simulink model "FaultCheck"  (R2022b)
settings: Solver=FixedStepAuto  StartTime=0.0  StopTime=10  FixedStep=1  RelTol=1e-3
undefined symbols (not defined in the file): C_Flt_IGBTULowerTempConfirmTh_u16, C_Flt_IGBTULowerTempDiagEn_b, C_Flt_IGBTULowerTempErrCode_u16, C_Flt_IGBTULowerTempPowerCoeff, C_Flt_IGBTULowerTempRecoveryTh_u16, C_Flt_IGBTULowerTempRecTh_s32, C_Flt_IGBTULowerTempTrigTh_s32, C_Flt_IGBTUOverTempConfirmTh_u16, C_Flt_IGBTUOverTempDiagEn_b, C_Flt_IGBTUOverTempErrCode_u16, C_Flt_IGBTUOverTempRecoveryTh_u16, C_Flt_IGBTUOverTempRecTh_s32, C_Flt_IGBTUOverTempTrigTh_s32, C_Flt_IGBTVLowerTempConfirmTh_u16, C_Flt_IGBTVLowerTempDiagEn_b, C_Flt_IGBTVLowerTempErrCode_u16, C_Flt_IGBTVLowerTempPowerCoeff, C_Flt_IGBTVLowerTempRecoveryTh_u16, C_Flt_IGBTVLowerTempRecTh_s32, C_Flt_IGBTVLowerTempTrigTh_s32, C_Flt_IGBTVOverTempConfirmTh_u16, C_Flt_IGBTVOverTempDiagEn_b, C_Flt_IGBTVOverTempErrCode_u16, C_Flt_IGBTVOverTempRecoveryTh_u16, C_Flt_IGBTVOverTempRecTh_s32, C_Flt_IGBTVOverTempTrigTh_s32, C_Flt_IGBTWLowerTempConfirmTh_u16, C_Flt_IGBTWLowerTempDiagEn_b, C_Flt_IGBTWLowerTempErrCode_u16, C_Flt_IGBTWLowerTempPowerCoeff, C_Flt_IGBTWLowerTempRecoveryTh_u16, C_Flt_IGBTWLowerTempRecTh_s32, C_Flt_IGBTWLowerTempTrigTh_s32, C_Flt_IGBTWOverTempConfirmTh_u16, C_Flt_IGBTWOverTempDiagEn_b, C_Flt_IGBTWOverTempErrCode_u16, C_Flt_IGBTWOverTempRecoveryTh_u16, C_Flt_IGBTWOverTempRecTh_s32, C_Flt_IGBTWOverTempTrigTh_s32, C_Flt_IuOCConfirmTh_u16, C_Flt_IuOCDiagEn_b, C_Flt_IuOCErrCode_u16, C_Flt_IuOCNegLimit_s32, C_Flt_IuOCPosLimit_s32, C_Flt_IuOCRecoveryTh_u16, C_Flt_IuZeroDriftDiagEn_b, C_Flt_IuZeroDriftErrCode_u16, C_Flt_IvOCConfirmTh_u16, C_Flt_IvOCDiagEn_b, C_Flt_IvOCErrCode_u16, C_Flt_IvOCNegLimit_s32, C_Flt_IvOCPosLimit_s32, C_Flt_IvOCRecoveryTh_u16, C_Flt_IvZeroDriftDiagEn_b, C_Flt_IvZeroDriftErrCode_u16, C_Flt_IwOCConfirmTh_u16, C_Flt_IwOCDiagEn_b, C_Flt_IwOCErrCode_u16, C_Flt_IwOCNegLimit_s32, C_Flt_IwOCPosLimit_s32 ... (+196)
libraries: YS_UserDefined_Library x21, simulink x5
(part 9 of 11)

== system FaultCheck/FaultDiag_HighTask_100us/FltDetn/CurrentSensorDetn/Flt_CurrentSensorDetn/ErrCode/If Action Subsystem ==
  Action Port : ActionPort
  Assignment : Assignment  IndexMode=Zero-based  DiagnosticForDimensions=Warning  IndexOptions=Index vector (port)  Indices=1  OutputSizes=1
  Constant : Constant  Value=FLT_ERRCODE_0  OutDataTypeStr=fixdt('uint16', 'DataTypeOverride', 'Off')
  Constant1 : Constant  Value=FLT_ERRBIT_53
  Data Store Read : DataStoreRead  DataStoreName=Flt_ErrCode  IndexOptions=Index vector (dialog)  Indices=1  OutputSizes=1
  Data Store Write : DataStoreWrite  DataStoreName=Flt_ErrCode  IndexOptions=Index vector (dialog)  Indices=1  OutputSizes=1
  wires:
  Assignment/1 -> Data Store Write/1
  Constant/1 -> Assignment/2
  Data Store Read/1 -> Assignment/1
  Constant1/1 -> Assignment/3

== system FaultCheck/FaultDiag_HighTask_100us/FltDetn/CurrentSensorDetn/Flt_CurrentSensorDetn/ErrCode/If Action Subsystem1 ==
  ErrCod : Inport
  Action Port : ActionPort
  Assignment : Assignment  IndexMode=Zero-based  DiagnosticForDimensions=Warning  IndexOptions=Index vector (port)  Indices=1  OutputSizes=1
  Constant : Constant  Value=FLT_ERRBIT_53
  Data Store Read : DataStoreRead  DataStoreName=Flt_ErrCode  IndexOptions=Index vector (dialog)  Indices=1  OutputSizes=1
  Data Store Write : DataStoreWrite  DataStoreName=Flt_ErrCode  IndexOptions=Index vector (dialog)  Indices=1  OutputSizes=1
  wires:
  Constant/1 -> Assignment/3
  ErrCod/1 -> Assignment/2
  Assignment/1 -> Data Store Write/1
  Data Store Read/1 -> Assignment/1

== system FaultCheck/FaultDiag_HighTask_100us/FltDetn/CurrentSensorDetn/Flt_CurrentSensorDetn/ErrDetn/If Action Subsystem ==
  Action Port : ActionPort
  Constant : Constant  Value=FLT_NOERR
  Out1 : Outport
  wires:
  Constant/1 -> Out1/1

== system FaultCheck/FaultDiag_HighTask_100us/FltDetn/CurrentSensorDetn/Flt_CurrentSensorDetn/ErrDetn/If Action Subsystem1 ==
  InputVal : Inport
  ErrDeb : Inport  Port=2
  Action Port : ActionPort
  Constant3 : Constant  Value=FLT_ERR
  Debounce1 : Subsystem
  Delay1 : Delay  DelayLength=1
  Signal Conversion : SignalConversion  OverrideOpt=off
  Switch2 : Switch  Criteria=u2 > Threshold  SaturateOnIntegerOverflow=off  InputSameDT=off
  Out1 : Outport
  wires:
  Signal Conversion/1 -> Out1/1
  Delay1/1 -> Switch2/3
  Constant3/1 -> Switch2/1
  Switch2/1 -> Signal Conversion/1, Delay1/1
  Debounce1/1(ErrFlg) -> Switch2/2
  InputVal/1 -> Debounce1/1(ErrInput)
  ErrDeb/1 -> Debounce1/2(ErrDeb)

== system FaultCheck/FaultDiag_HighTask_100us/FltDetn/CurrentSensorDetn/Flt_CurrentSensorDetn/FltLvl/If Action Subsystem ==
  Action Port : ActionPort
  Constant : Constant  Value=FLTLVL_ZERO
  ValOut : Outport
  wires:
  Constant/1 -> ValOut/1

== system FaultCheck/FaultDiag_HighTask_100us/FltDetn/CurrentSensorDetn/Flt_CurrentSensorDetn/FltLvl/If Action Subsystem1 ==
  In : Inport
  Action Port : ActionPort
  ValOut : Outport
  wires:
  In/1 -> ValOut/1

== system FaultCheck/FaultDiag_HighTask_100us/FltDetn/CurrentSensorDetn/Flt_CurrentSensorDetn/Power Reduction Coefficient/If Action Subsystem ==
  Action Port : ActionPort
  Constant1 : Constant  Value=FLT_COEF_ONE
  PowRecCoefOut : Outport
  wires:
  Constant1/1 -> PowRecCoefOut/1

== system FaultCheck/FaultDiag_HighTask_100us/FltDetn/CurrentSensorDetn/Flt_CurrentSensorDetn/Power Reduction Coefficient/If Action Subsystem1 ==
  PowRecCoef : Inport
  Action Port : ActionPort
  PowRecCoefOut : Outport
  wires:
  PowRecCoef/1 -> PowRecCoefOut/1

== system FaultCheck/FaultDiag_HighTask_100us/FltDetn/CurrentSensorDetn/Flt_CurrentSensorDetn/Power Reduction Coefficient/If Action Subsystem2 ==
  Action Port : ActionPort
  Constant1 : Constant  Value=FLT_COEF_ZERO
  PowRecCoefOut : Outport
  wires:
  Constant1/1 -> PowRecCoefOut/1

== system FaultCheck/FaultDiag_HighTask_100us/FltDetn/CurrentZeroDrfDetn/CurrZeroDrfDetn/ErrCode1/If Action Subsystem ==
  Action Port : ActionPort
  Assignment : Assignment  IndexMode=Zero-based  DiagnosticForDimensions=Warning  IndexOptions=Index vector (port)  Indices=1  OutputSizes=1
  Constant : Constant  Value=FLT_ERRCODE_0
  Constant1 : Constant  Value=FLT_ERRBIT_55
  Data Store Read : DataStoreRead  DataStoreName=Flt_ErrCode  IndexOptions=Index vector (dialog)  Indices=1  OutputSizes=1
  Data Store Write : DataStoreWrite  DataStoreName=Flt_ErrCode  IndexOptions=Index vector (dialog)  Indices=1  OutputSizes=1
  wires:
  Constant1/1 -> Assignment/3
  Data Store Read/1 -> Assignment/1
  Constant/1 -> Assignment/2
  Assignment/1 -> Data Store Write/1

== system FaultCheck/FaultDiag_HighTask_100us/FltDetn/CurrentZeroDrfDetn/CurrZeroDrfDetn/ErrCode1/If Action Subsystem1 ==
  ErrCod : Inport
  Action Port : ActionPort
  Assignment : Assignment  IndexMode=Zero-based  DiagnosticForDimensions=Warning  IndexOptions=Index vector (port)  Indices=1  OutputSizes=1
  Constant : Constant  Value=FLT_ERRBIT_55
  Data Store Read : DataStoreRead  DataStoreName=Flt_ErrCode  IndexOptions=Index vector (dialog)  Indices=1  OutputSizes=1
  Data Store Write : DataStoreWrite  DataStoreName=Flt_ErrCode  IndexOptions=Index vector (dialog)  Indices=1  OutputSizes=1
  wires:
  Data Store Read/1 -> Assignment/1
  Assignment/1 -> Data Store Write/1
  ErrCod/1 -> Assignment/2
  Constant/1 -> Assignment/3

== system FaultCheck/FaultDiag_HighTask_100us/FltDetn/CurrentZeroDrfDetn/CurrZeroDrfDetn/ErrDetn/If Action Subsystem ==
  Action Port : ActionPort
  Constant : Constant  Value=FLT_NOERR
  Out1 : Outport
  wires:
  Constant/1 -> Out1/1

== system FaultCheck/FaultDiag_HighTask_100us/FltDetn/CurrentZeroDrfDetn/CurrZeroDrfDetn/ErrDetn/If Action Subsystem1 ==
  InputVal : Inport
  Action Port : ActionPort
  Constant3 : Constant  Value=FLT_ERR
  Delay1 : Delay  DelayLength=1
  Switch2 : Switch  Criteria=u2 > Threshold  SaturateOnIntegerOverflow=off  InputSameDT=off
  Out1 : Outport
  wires:
  Delay1/1 -> Switch2/3
  Constant3/1 -> Switch2/1
  Switch2/1 -> Out1/1, Delay1/1
  InputVal/1 -> Switch2/2

== system FaultCheck/FaultDiag_HighTask_100us/FltDetn/CurrentZeroDrfDetn/CurrZeroDrfDetn/FltLvl/If Action Subsystem ==
  Action Port : ActionPort
  Constant : Constant  Value=FLTLVL_ZERO
  ValOut : Outport
  wires:
  Constant/1 -> ValOut/1

== system FaultCheck/FaultDiag_HighTask_100us/FltDetn/CurrentZeroDrfDetn/CurrZeroDrfDetn/FltLvl/If Action Subsystem1 ==
  In : Inport
  Action Port : ActionPort
  ValOut : Outport
  wires:
  In/1 -> ValOut/1

== system FaultCheck/FaultDiag_HighTask_100us/FltDetn/CurrentZeroDrfDetn/CurrZeroDrfDetn/Power Reduction Coefficient/If Action Subsystem ==
  Action Port : ActionPort
  Constant1 : Constant  Value=FLT_COEF_ONE
  PowRecCoefOut : Outport
  wires:
  Constant1/1 -> PowRecCoefOut/1

== system FaultCheck/FaultDiag_HighTask_100us/FltDetn/CurrentZeroDrfDetn/CurrZeroDrfDetn/Power Reduction Coefficient/If Action Subsystem1 ==
  PowRecCoef : Inport
  Action Port : ActionPort
  PowRecCoefOut : Outport
  wires:
  PowRecCoef/1 -> PowRecCoefOut/1

== system FaultCheck/FaultDiag_HighTask_100us/FltDetn/CurrentZeroDrfDetn/CurrZeroDrfDetn/Power Reduction Coefficient/If Action Subsystem2 ==
  Action Port : ActionPort
  Constant1 : Constant  Value=FLT_COEF_ZERO
  PowRecCoefOut : Outport
  wires:
  Constant1/1 -> PowRecCoefOut/1

== system FaultCheck/FaultDiag_HighTask_100us/FltDetn/DriveUdcDetn/DriveUdcDetn/ErrCode/If Action Subsystem ==
  Action Port : ActionPort
  Assignment : Assignment  IndexMode=Zero-based  DiagnosticForDimensions=Warning  IndexOptions=Index vector (port)  Indices=1  OutputSizes=1
  Constant : Constant  Value=FLT_ERRCODE_0
  Constant1 : Constant  Value=FLT_ERRBIT_53
  Data Store Read : DataStoreRead  DataStoreName=Flt_ErrCode  IndexOptions=Index vector (dialog)  Indices=1  OutputSizes=1
  Data Store Write : DataStoreWrite  DataStoreName=Flt_ErrCode  IndexOptions=Index vector (dialog)  Indices=1  OutputSizes=1
  wires:
  Constant1/1 -> Assignment/3
  Data Store Read/1 -> Assignment/1
  Constant/1 -> Assignment/2
  Assignment/1 -> Data Store Write/1

== system FaultCheck/FaultDiag_HighTask_100us/FltDetn/DriveUdcDetn/DriveUdcDetn/ErrCode/If Action Subsystem1 ==
  ErrCod : Inport
  Action Port : ActionPort
  Assignment : Assignment  IndexMode=Zero-based  DiagnosticForDimensions=Warning  IndexOptions=Index vector (port)  Indices=1  OutputSizes=1
  Constant : Constant  Value=FLT_ERRBIT_53
  Data Store Read : DataStoreRead  DataStoreName=Flt_ErrCode  IndexOptions=Index vector (dialog)  Indices=1  OutputSizes=1
  Data Store Write : DataStoreWrite  DataStoreName=Flt_ErrCode  IndexOptions=Index vector (dialog)  Indices=1  OutputSizes=1
  wires:
  Data Store Read/1 -> Assignment/1
  Assignment/1 -> Data Store Write/1
  ErrCod/1 -> Assignment/2
  Constant/1 -> Assignment/3

== system FaultCheck/FaultDiag_HighTask_100us/FltDetn/DriveUdcDetn/DriveUdcDetn/ErrDetn/If Action Subsystem ==
  Action Port : ActionPort
  Constant : Constant  Value=FLT_NOERR
  Out1 : Outport
  wires:
  Constant/1 -> Out1/1

== system FaultCheck/FaultDiag_HighTask_100us/FltDetn/DriveUdcDetn/DriveUdcDetn/ErrDetn/If Action Subsystem1 ==
  InputVal : Inport
  ErrDeb : Inport  Port=2
  Action Port : ActionPort
  Constant3 : Constant  Value=FLT_ERR
  Debounce1 : Subsystem
  Delay1 : Delay  DelayLength=1
  Switch2 : Switch  Criteria=u2 > Threshold  SaturateOnIntegerOverflow=off  InputSameDT=off
  Out1 : Outport
  wires:
  ErrDeb/1 -> Debounce1/2(ErrDeb)
  InputVal/1 -> Debounce1/1(ErrInput)
  Debounce1/1(ErrFlg) -> Switch2/2
  Switch2/1 -> Delay1/1, Out1/1
  Constant3/1 -> Switch2/1
  Delay1/1 -> Switch2/3

== system FaultCheck/FaultDiag_HighTask_100us/FltDetn/DriveUdcDetn/DriveUdcDetn/FltLvl/If Action Subsystem ==
  Action Port : ActionPort
  Constant : Constant  Value=FLTLVL_ZERO
  ValOut : Outport
  wires:
  Constant/1 -> ValOut/1

== system FaultCheck/FaultDiag_HighTask_100us/FltDetn/DriveUdcDetn/DriveUdcDetn/FltLvl/If Action Subsystem1 ==
  In : Inport
  Action Port : ActionPort
  ValOut : Outport
  wires:
  In/1 -> ValOut/1

== system FaultCheck/FaultDiag_HighTask_100us/FltDetn/DriveUdcDetn/DriveUdcDetn/Power Reduction Coefficient/If Action Subsystem ==
  Action Port : ActionPort
  Constant1 : Constant  Value=FLT_COEF_ONE
  PowRecCoefOut : Outport
  wires:
  Constant1/1 -> PowRecCoefOut/1

== system FaultCheck/FaultDiag_HighTask_100us/FltDetn/DriveUdcDetn/DriveUdcDetn/Power Reduction Coefficient/If Action Subsystem1 ==
  PowRecCoef : Inport
  Action Port : ActionPort
  PowRecCoefOut : Outport
  wires:
  PowRecCoef/1 -> PowRecCoefOut/1

== system FaultCheck/FaultDiag_HighTask_100us/FltDetn/DriveUdcDetn/DriveUdcDetn/Power Reduction Coefficient/If Action Subsystem2 ==
  Action Port : ActionPort
  Constant1 : Constant  Value=FLT_COEF_ZERO
  PowRecCoefOut : Outport
  wires:
  Constant1/1 -> PowRecCoefOut/1

== system FaultCheck/FaultDiag_HighTask_100us/FltDetn/Drive_H_Detn/Drive_H_Detn/ErrCode/If Action Subsystem ==
  Action Port : ActionPort
  Assignment : Assignment  IndexMode=Zero-based  DiagnosticForDimensions=Warning  IndexOptions=Index vector (port)  Indices=1  OutputSizes=1
  Constant : Constant  Value=FLT_ERRCODE_0
  Constant1 : Constant  Value=FLT_ERRBIT_53
  Data Store Read : DataStoreRead  DataStoreName=Flt_ErrCode  IndexOptions=Index vector (dialog)  Indices=1  OutputSizes=1
  Data Store Write : DataStoreWrite  DataStoreName=Flt_ErrCode  IndexOptions=Index vector (dialog)  Indices=1  OutputSizes=1
  wires:
  Constant1/1 -> Assignment/3
  Data Store Read/1 -> Assignment/1
  Constant/1 -> Assignment/2
  Assignment/1 -> Data Store Write/1

== system FaultCheck/FaultDiag_HighTask_100us/FltDetn/Drive_H_Detn/Drive_H_Detn/ErrCode/If Action Subsystem1 ==
  ErrCod : Inport
  Action Port : ActionPort
  Assignment : Assignment  IndexMode=Zero-based  DiagnosticForDimensions=Warning  IndexOptions=Index vector (port)  Indices=1  OutputSizes=1
  Constant : Constant  Value=FLT_ERRBIT_53
  Data Store Read : DataStoreRead  DataStoreName=Flt_ErrCode  IndexOptions=Index vector (dialog)  Indices=1  OutputSizes=1
  Data Store Write : DataStoreWrite  DataStoreName=Flt_ErrCode  IndexOptions=Index vector (dialog)  Indices=1  OutputSizes=1
  wires:
  Data Store Read/1 -> Assignment/1
  Assignment/1 -> Data Store Write/1
  ErrCod/1 -> Assignment/2
  Constant/1 -> Assignment/3

== system FaultCheck/FaultDiag_HighTask_100us/FltDetn/Drive_H_Detn/Drive_H_Detn/ErrDetn/If Action Subsystem ==
  Action Port : ActionPort
  Constant : Constant  Value=FLT_NOERR
  Out1 : Outport
  wires:
  Constant/1 -> Out1/1

== system FaultCheck/FaultDiag_HighTask_100us/FltDetn/Drive_H_Detn/Drive_H_Detn/ErrDetn/If Action Subsystem1 ==
  InputVal : Inport
  ErrDeb : Inport  Port=2
  Action Port : ActionPort
  Constant3 : Constant  Value=FLT_ERR
  Debounce1 : Subsystem
  Delay1 : Delay  DelayLength=1
  Switch2 : Switch  Criteria=u2 > Threshold  SaturateOnIntegerOverflow=off  InputSameDT=off
  Out1 : Outport
  wires:
  ErrDeb/1 -> Debounce1/2(ErrDeb)
  InputVal/1 -> Debounce1/1(ErrInput)
  Debounce1/1(ErrFlg) -> Switch2/2
  Switch2/1 -> Delay1/1, Out1/1
  Constant3/1 -> Switch2/1
  Delay1/1 -> Switch2/3

== system FaultCheck/FaultDiag_HighTask_100us/FltDetn/Drive_H_Detn/Drive_H_Detn/FltLvl/If Action Subsystem ==
  Action Port : ActionPort
  Constant : Constant  Value=FLTLVL_ZERO
  ValOut : Outport
  wires:
  Constant/1 -> ValOut/1

== system FaultCheck/FaultDiag_HighTask_100us/FltDetn/Drive_H_Detn/Drive_H_Detn/FltLvl/If Action Subsystem1 ==
  In : Inport
  Action Port : ActionPort
  ValOut : Outport
  wires:
  In/1 -> ValOut/1

== system FaultCheck/FaultDiag_HighTask_100us/FltDetn/Drive_H_Detn/Drive_H_Detn/Power Reduction Coefficient/If Action Subsystem ==
  Action Port : ActionPort
  Constant1 : Constant  Value=FLT_COEF_ONE
  PowRecCoefOut : Outport
  wires:
  Constant1/1 -> PowRecCoefOut/1

== system FaultCheck/FaultDiag_HighTask_100us/FltDetn/Drive_H_Detn/Drive_H_Detn/Power Reduction Coefficient/If Action Subsystem1 ==
  PowRecCoef : Inport
  Action Port : ActionPort
  PowRecCoefOut : Outport
  wires:
  PowRecCoef/1 -> PowRecCoefOut/1

== system FaultCheck/FaultDiag_HighTask_100us/FltDetn/Drive_H_Detn/Drive_H_Detn/Power Reduction Coefficient/If Action Subsystem2 ==
  Action Port : ActionPort
  Constant1 : Constant  Value=FLT_COEF_ZERO
  PowRecCoefOut : Outport
  wires:
  Constant1/1 -> PowRecCoefOut/1

== system FaultCheck/FaultDiag_HighTask_100us/FltDetn/Drive_L_Detn/Drive_L_Detn/ErrCode/If Action Subsystem ==
  Action Port : ActionPort
  Assignment : Assignment  IndexMode=Zero-based  DiagnosticForDimensions=Warning  IndexOptions=Index vector (port)  Indices=1  OutputSizes=1
  Constant : Constant  Value=FLT_ERRCODE_0
  Constant1 : Constant  Value=FLT_ERRBIT_53
  Data Store Read : DataStoreRead  DataStoreName=Flt_ErrCode  IndexOptions=Index vector (dialog)  Indices=1  OutputSizes=1
  Data Store Write : DataStoreWrite  DataStoreName=Flt_ErrCode  IndexOptions=Index vector (dialog)  Indices=1  OutputSizes=1
  wires:
  Constant1/1 -> Assignment/3
  Data Store Read/1 -> Assignment/1
  Constant/1 -> Assignment/2
  Assignment/1 -> Data Store Write/1

== system FaultCheck/FaultDiag_HighTask_100us/FltDetn/Drive_L_Detn/Drive_L_Detn/ErrCode/If Action Subsystem1 ==
  ErrCod : Inport
  Action Port : ActionPort
  Assignment : Assignment  IndexMode=Zero-based  DiagnosticForDimensions=Warning  IndexOptions=Index vector (port)  Indices=1  OutputSizes=1
  Constant : Constant  Value=FLT_ERRBIT_53
  Data Store Read : DataStoreRead  DataStoreName=Flt_ErrCode  IndexOptions=Index vector (dialog)  Indices=1  OutputSizes=1
  Data Store Write : DataStoreWrite  DataStoreName=Flt_ErrCode  IndexOptions=Index vector (dialog)  Indices=1  OutputSizes=1
  wires:
  Data Store Read/1 -> Assignment/1
  Assignment/1 -> Data Store Write/1
  ErrCod/1 -> Assignment/2
  Constant/1 -> Assignment/3

== system FaultCheck/FaultDiag_HighTask_100us/FltDetn/Drive_L_Detn/Drive_L_Detn/ErrDetn/If Action Subsystem ==
  Action Port : ActionPort
  Constant : Constant  Value=FLT_NOERR
  Out1 : Outport
  wires:
  Constant/1 -> Out1/1

== system FaultCheck/FaultDiag_HighTask_100us/FltDetn/Drive_L_Detn/Drive_L_Detn/ErrDetn/If Action Subsystem1 ==
  InputVal : Inport
  ErrDeb : Inport  Port=2
  Action Port : ActionPort
  Constant3 : Constant  Value=FLT_ERR
  Debounce1 : Subsystem
  Delay1 : Delay  DelayLength=1
  Switch2 : Switch  Criteria=u2 > Threshold  SaturateOnIntegerOverflow=off  InputSameDT=off
  Out1 : Outport
  wires:
  ErrDeb/1 -> Debounce1/2(ErrDeb)
  InputVal/1 -> Debounce1/1(ErrInput)
  Debounce1/1(ErrFlg) -> Switch2/2
  Switch2/1 -> Delay1/1, Out1/1
  Constant3/1 -> Switch2/1
  Delay1/1 -> Switch2/3

== system FaultCheck/FaultDiag_HighTask_100us/FltDetn/Drive_L_Detn/Drive_L_Detn/FltLvl/If Action Subsystem ==
  Action Port : ActionPort
  Constant : Constant  Value=FLTLVL_ZERO
  ValOut : Outport
  wires:
  Constant/1 -> ValOut/1

== system FaultCheck/FaultDiag_HighTask_100us/FltDetn/Drive_L_Detn/Drive_L_Detn/FltLvl/If Action Subsystem1 ==
  In : Inport
  Action Port : ActionPort
  ValOut : Outport
  wires:
  In/1 -> ValOut/1

== system FaultCheck/FaultDiag_HighTask_100us/FltDetn/Drive_L_Detn/Drive_L_Detn/Power Reduction Coefficient/If Action Subsystem ==
  Action Port : ActionPort
  Constant1 : Constant  Value=FLT_COEF_ONE
  PowRecCoefOut : Outport
  wires:
  Constant1/1 -> PowRecCoefOut/1

== system FaultCheck/FaultDiag_HighTask_100us/FltDetn/Drive_L_Detn/Drive_L_Detn/Power Reduction Coefficient/If Action Subsystem1 ==
  PowRecCoef : Inport
  Action Port : ActionPort
  PowRecCoefOut : Outport
  wires:
  PowRecCoef/1 -> PowRecCoefOut/1

== system FaultCheck/FaultDiag_HighTask_100us/FltDetn/Drive_L_Detn/Drive_L_Detn/Power Reduction Coefficient/If Action Subsystem2 ==
  Action Port : ActionPort
  Constant1 : Constant  Value=FLT_COEF_ZERO
  PowRecCoefOut : Outport
  wires:
  Constant1/1 -> PowRecCoefOut/1

== system FaultCheck/FaultDiag_HighTask_100us/FltDetn/HWOverCurrDetn/HWOverCurrDetn/ErrCode/If Action Subsystem ==
  Action Port : ActionPort
  Assignment : Assignment  IndexMode=Zero-based  DiagnosticForDimensions=Warning  IndexOptions=Index vector (port)  Indices=1  OutputSizes=1
  Constant : Constant  Value=FLT_ERRCODE_0
  Constant1 : Constant  Value=FLT_ERRBIT_53
  Data Store Read : DataStoreRead  DataStoreName=Flt_ErrCode  IndexOptions=Index vector (dialog)  Indices=1  OutputSizes=1
  Data Store Write : DataStoreWrite  DataStoreName=Flt_ErrCode  IndexOptions=Index vector (dialog)  Indices=1  OutputSizes=1
  wires:
  Constant1/1 -> Assignment/3
  Data Store Read/1 -> Assignment/1
  Constant/1 -> Assignment/2
  Assignment/1 -> Data Store Write/1

== system FaultCheck/FaultDiag_HighTask_100us/FltDetn/HWOverCurrDetn/HWOverCurrDetn/ErrCode/If Action Subsystem1 ==
  ErrCod : Inport
  Action Port : ActionPort
  Assignment : Assignment  IndexMode=Zero-based  DiagnosticForDimensions=Warning  IndexOptions=Index vector (port)  Indices=1  OutputSizes=1
  Constant : Constant  Value=FLT_ERRBIT_53
  Data Store Read : DataStoreRead  DataStoreName=Flt_ErrCode  IndexOptions=Index vector (dialog)  Indices=1  OutputSizes=1
  Data Store Write : DataStoreWrite  DataStoreName=Flt_ErrCode  IndexOptions=Index vector (dialog)  Indices=1  OutputSizes=1
  wires:
  Data Store Read/1 -> Assignment/1
  Assignment/1 -> Data Store Write/1
  ErrCod/1 -> Assignment/2
  Constant/1 -> Assignment/3

== system FaultCheck/FaultDiag_HighTask_100us/FltDetn/HWOverCurrDetn/HWOverCurrDetn/ErrDetn/If Action Subsystem ==
  Action Port : ActionPort
  Constant : Constant  Value=FLT_NOERR
  Out1 : Outport
  wires:
  Constant/1 -> Out1/1

== system FaultCheck/FaultDiag_HighTask_100us/FltDetn/HWOverCurrDetn/HWOverCurrDetn/ErrDetn/If Action Subsystem1 ==
  InputVal : Inport
  ErrDeb : Inport  Port=2
  Action Port : ActionPort
  Constant3 : Constant  Value=FLT_ERR
  Debounce1 : Subsystem
  Delay1 : Delay  DelayLength=1
  Switch2 : Switch  Criteria=u2 > Threshold  SaturateOnIntegerOverflow=off  InputSameDT=off
  Out1 : Outport
  wires:
  ErrDeb/1 -> Debounce1/2(ErrDeb)
  InputVal/1 -> Debounce1/1(ErrInput)
  Debounce1/1(ErrFlg) -> Switch2/2
  Switch2/1 -> Delay1/1, Out1/1
  Constant3/1 -> Switch2/1
  Delay1/1 -> Switch2/3

== system FaultCheck/FaultDiag_HighTask_100us/FltDetn/HWOverCurrDetn/HWOverCurrDetn/FltLvl/If Action Subsystem ==
  Action Port : ActionPort
  Constant : Constant  Value=FLTLVL_ZERO
  ValOut : Outport
  wires:
  Constant/1 -> ValOut/1

== system FaultCheck/FaultDiag_HighTask_100us/FltDetn/HWOverCurrDetn/HWOverCurrDetn/FltLvl/If Action Subsystem1 ==
  In : Inport
  Action Port : ActionPort
  ValOut : Outport
  wires:
  In/1 -> ValOut/1

== system FaultCheck/FaultDiag_HighTask_100us/FltDetn/HWOverCurrDetn/HWOverCurrDetn/Power Reduction Coefficient/If Action Subsystem ==
  Action Port : ActionPort
  Constant1 : Constant  Value=FLT_COEF_ONE
  PowRecCoefOut : Outport
  wires:
  Constant1/1 -> PowRecCoefOut/1

== system FaultCheck/FaultDiag_HighTask_100us/FltDetn/HWOverCurrDetn/HWOverCurrDetn/Power Reduction Coefficient/If Action Subsystem1 ==
  PowRecCoef : Inport
  Action Port : ActionPort
  PowRecCoefOut : Outport
  wires:
  PowRecCoef/1 -> PowRecCoefOut/1

== system FaultCheck/FaultDiag_HighTask_100us/FltDetn/HWOverCurrDetn/HWOverCurrDetn/Power Reduction Coefficient/If Action Subsystem2 ==
  Action Port : ActionPort
  Constant1 : Constant  Value=FLT_COEF_ZERO
  PowRecCoefOut : Outport
  wires:
  Constant1/1 -> PowRecCoefOut/1

== system FaultCheck/FaultDiag_HighTask_100us/FltDetn/HWOverUdcDetn/HWOverCurrDetn/ErrCode/If Action Subsystem ==
  Action Port : ActionPort
  Assignment : Assignment  IndexMode=Zero-based  DiagnosticForDimensions=Warning  IndexOptions=Index vector (port)  Indices=1  OutputSizes=1
  Constant : Constant  Value=FLT_ERRCODE_0
  Constant1 : Constant  Value=FLT_ERRBIT_53
  Data Store Read : DataStoreRead  DataStoreName=Flt_ErrCode  IndexOptions=Index vector (dialog)  Indices=1  OutputSizes=1
  Data Store Write : DataStoreWrite  DataStoreName=Flt_ErrCode  IndexOptions=Index vector (dialog)  Indices=1  OutputSizes=1
  wires:
  Constant1/1 -> Assignment/3
  Data Store Read/1 -> Assignment/1
  Constant/1 -> Assignment/2
  Assignment/1 -> Data Store Write/1

== system FaultCheck/FaultDiag_HighTask_100us/FltDetn/HWOverUdcDetn/HWOverCurrDetn/ErrCode/If Action Subsystem1 ==
  ErrCod : Inport
  Action Port : ActionPort
  Assignment : Assignment  IndexMode=Zero-based  DiagnosticForDimensions=Warning  IndexOptions=Index vector (port)  Indices=1  OutputSizes=1
  Constant : Constant  Value=FLT_ERRBIT_53
  Data Store Read : DataStoreRead  DataStoreName=Flt_ErrCode  IndexOptions=Index vector (dialog)  Indices=1  OutputSizes=1
  Data Store Write : DataStoreWrite  DataStoreName=Flt_ErrCode  IndexOptions=Index vector (dialog)  Indices=1  OutputSizes=1
  wires:
  Data Store Read/1 -> Assignment/1
  Assignment/1 -> Data Store Write/1
  ErrCod/1 -> Assignment/2
  Constant/1 -> Assignment/3

== system FaultCheck/FaultDiag_HighTask_100us/FltDetn/HWOverUdcDetn/HWOverCurrDetn/ErrDetn/If Action Subsystem ==
  Action Port : ActionPort
  Constant : Constant  Value=FLT_NOERR
  Out1 : Outport
  wires:
  Constant/1 -> Out1/1

== system FaultCheck/FaultDiag_HighTask_100us/FltDetn/HWOverUdcDetn/HWOverCurrDetn/ErrDetn/If Action Subsystem1 ==
  InputVal : Inport
  ErrDeb : Inport  Port=2
  Action Port : ActionPort
  Constant3 : Constant  Value=FLT_ERR
  Debounce1 : Subsystem
  Delay1 : Delay  DelayLength=1
  Switch2 : Switch  Criteria=u2 > Threshold  SaturateOnIntegerOverflow=off  InputSameDT=off
  Out1 : Outport
  wires:
  ErrDeb/1 -> Debounce1/2(ErrDeb)
  InputVal/1 -> Debounce1/1(ErrInput)
  Debounce1/1(ErrFlg) -> Switch2/2
  Switch2/1 -> Delay1/1, Out1/1
  Constant3/1 -> Switch2/1
  Delay1/1 -> Switch2/3

== system FaultCheck/FaultDiag_HighTask_100us/FltDetn/HWOverUdcDetn/HWOverCurrDetn/FltLvl/If Action Subsystem ==
  Action Port : ActionPort
  Constant : Constant  Value=FLTLVL_ZERO
  ValOut : Outport
  wires:
  Constant/1 -> ValOut/1

== system FaultCheck/FaultDiag_HighTask_100us/FltDetn/HWOverUdcDetn/HWOverCurrDetn/FltLvl/If Action Subsystem1 ==
  In : Inport
  Action Port : ActionPort
  ValOut : Outport
  wires:
  In/1 -> ValOut/1

== system FaultCheck/FaultDiag_HighTask_100us/FltDetn/HWOverUdcDetn/HWOverCurrDetn/Power Reduction Coefficient/If Action Subsystem ==
  Action Port : ActionPort
  Constant1 : Constant  Value=FLT_COEF_ONE
  PowRecCoefOut : Outport
  wires:
  Constant1/1 -> PowRecCoefOut/1

== system FaultCheck/FaultDiag_HighTask_100us/FltDetn/HWOverUdcDetn/HWOverCurrDetn/Power Reduction Coefficient/If Action Subsystem1 ==
  PowRecCoef : Inport
  Action Port : ActionPort
  PowRecCoefOut : Outport
  wires:
  PowRecCoef/1 -> PowRecCoefOut/1

== system FaultCheck/FaultDiag_HighTask_100us/FltDetn/HWOverUdcDetn/HWOverCurrDetn/Power Reduction Coefficient/If Action Subsystem2 ==
  Action Port : ActionPort
  Constant1 : Constant  Value=FLT_COEF_ZERO
  PowRecCoefOut : Outport
  wires:
  Constant1/1 -> PowRecCoefOut/1

== system FaultCheck/FaultDiag_HighTask_100us/FltDetn/OverCurrDetn/Flt_IuOverCurrDetn/ErrCode1/If Action Subsystem ==
  Action Port : ActionPort
  Assignment : Assignment  IndexMode=Zero-based  DiagnosticForDimensions=Warning  IndexOptions=Index vector (port)  Indices=1  OutputSizes=1
  Constant : Constant  Value=FLT_ERRCODE_0
  Constant1 : Constant  Value=FLT_ERRBIT_50
  Data Store Read : DataStoreRead  DataStoreName=Flt_ErrCode  IndexOptions=Index vector (dialog)  Indices=1  OutputSizes=1
  Data Store Write : DataStoreWrite  DataStoreName=Flt_ErrCode  IndexOptions=Index vector (dialog)  Indices=1  OutputSizes=1
  wires:
  Constant1/1 -> Assignment/3
  Data Store Read/1 -> Assignment/1
  Constant/1 -> Assignment/2
  Assignment/1 -> Data Store Write/1

== system FaultCheck/FaultDiag_HighTask_100us/FltDetn/OverCurrDetn/Flt_IuOverCurrDetn/ErrCode1/If Action Subsystem1 ==
  ErrCod : Inport
  Action Port : ActionPort
  Assignment : Assignment  IndexMode=Zero-based  DiagnosticForDimensions=Warning  IndexOptions=Index vector (port)  Indices=1  OutputSizes=1
  Constant : Constant  Value=FLT_ERRBIT_50
  Data Store Read : DataStoreRead  DataStoreName=Flt_ErrCode  IndexOptions=Index vector (dialog)  Indices=1  OutputSizes=1
  Data Store Write : DataStoreWrite  DataStoreName=Flt_ErrCode  IndexOptions=Index vector (dialog)  Indices=1  OutputSizes=1
  wires:
  Data Store Read/1 -> Assignment/1
  Assignment/1 -> Data Store Write/1
  ErrCod/1 -> Assignment/2
  Constant/1 -> Assignment/3

== system FaultCheck/FaultDiag_HighTask_100us/FltDetn/OverCurrDetn/Flt_IuOverCurrDetn/ErrDetn1/If Action Subsystem ==
  Action Port : ActionPort
  Constant : Constant  Value=FLT_NOERR
  DetnFlg : Outport
  wires:
  Constant/1 -> DetnFlg/1

== system FaultCheck/FaultDiag_HighTask_100us/FltDetn/OverCurrDetn/Flt_IuOverCurrDetn/ErrDetn1/If Action Subsystem1 ==
  InputVal : Inport
  ErrDeb : Inport  Port=2
  HiLimPositv : Inport  Port=3
  HiLimNegatv : Inport  Port=4
  Action Port : ActionPort
  Constant3 : Constant  Value=FLT_ERR
  Debounce1 : Subsystem
  Delay1 : Delay  DelayLength=1
  OR : Logic  Operator=OR  AllPortsSameDT=off  OutDataTypeStr=boolean
  Relational Operator : RelationalOperator  Operator=<=  OutDataTypeStr=boolean  RndMeth=Simplest  InputSameDT=off
  Relational Operator1 : RelationalOperator  OutDataTypeStr=boolean  RndMeth=Simplest  InputSameDT=off
  Switch2 : Switch  Criteria=u2 > Threshold  SaturateOnIntegerOverflow=off  InputSameDT=off
  DetnFlg : Outport  PortDimensions=1
  wires:
  ErrDeb/1 -> Debounce1/2(ErrDeb)
  Debounce1/1(ErrFlg) -> Switch2/2
  Switch2/1 -> DetnFlg/1, Delay1/1
  Constant3/1 -> Switch2/1
  Delay1/1 -> Switch2/3
  HiLimNegatv/1 -> Relational Operator/2
  OR/1 -> Debounce1/1(ErrInput)
  HiLimPositv/1 -> Relational Operator1/2
  Relational Operator1/1 -> OR/1
  Relational Operator/1 -> OR/2
  InputVal/1 -> Relational Operator/1, Relational Operator1/1

== system FaultCheck/FaultDiag_HighTask_100us/FltDetn/OverCurrDetn/Flt_IuOverCurrDetn/FltLvl/If Action Subsystem ==
  Action Port : ActionPort
  Constant : Constant  Value=FLTLVL_ZERO
  ValOut : Outport
  wires:
  Constant/1 -> ValOut/1

== system FaultCheck/FaultDiag_HighTask_100us/FltDetn/OverCurrDetn/Flt_IuOverCurrDetn/FltLvl/If Action Subsystem1 ==
  In : Inport
  Action Port : ActionPort
  ValOut : Outport
  wires:
  In/1 -> ValOut/1

== system FaultCheck/FaultDiag_HighTask_100us/FltDetn/OverCurrDetn/Flt_IuOverCurrDetn/Power Reduction Coefficient/If Action Subsystem ==
  Action Port : ActionPort
  Constant1 : Constant  Value=FLT_COEF_ONE
  PowRecCoefOut : Outport
  wires:
  Constant1/1 -> PowRecCoefOut/1

== system FaultCheck/FaultDiag_HighTask_100us/FltDetn/OverCurrDetn/Flt_IuOverCurrDetn/Power Reduction Coefficient/If Action Subsystem1 ==
  PowRecCoef : Inport
  Action Port : ActionPort
  PowRecCoefOut : Outport
  wires:
  PowRecCoef/1 -> PowRecCoefOut/1

== system FaultCheck/FaultDiag_HighTask_100us/FltDetn/OverCurrDetn/Flt_IuOverCurrDetn/Power Reduction Coefficient/If Action Subsystem2 ==
  Action Port : ActionPort
  Constant1 : Constant  Value=FLT_COEF_ZERO
  PowRecCoefOut : Outport
  wires:
  Constant1/1 -> PowRecCoefOut/1

== system FaultCheck/FaultDiag_HighTask_100us/FltDetn/OverCurrDetn/Flt_IvOverCurrDetn/ErrCode1/If Action Subsystem ==
  Action Port : ActionPort
  Assignment : Assignment  IndexMode=Zero-based  DiagnosticForDimensions=Warning  IndexOptions=Index vector (port)  Indices=1  OutputSizes=1
  Constant : Constant  Value=FLT_ERRCODE_0
  Constant1 : Constant  Value=FLT_ERRBIT_51
  Data Store Read : DataStoreRead  DataStoreName=Flt_ErrCode  IndexOptions=Index vector (dialog)  Indices=1  OutputSizes=1
  Data Store Write : DataStoreWrite  DataStoreName=Flt_ErrCode  IndexOptions=Index vector (dialog)  Indices=1  OutputSizes=1
  wires:
  Constant1/1 -> Assignment/3
  Data Store Read/1 -> Assignment/1
  Constant/1 -> Assignment/2
  Assignment/1 -> Data Store Write/1

== system FaultCheck/FaultDiag_HighTask_100us/FltDetn/OverCurrDetn/Flt_IvOverCurrDetn/ErrCode1/If Action Subsystem1 ==
  ErrCod : Inport
  Action Port : ActionPort
  Assignment : Assignment  IndexMode=Zero-based  DiagnosticForDimensions=Warning  IndexOptions=Index vector (port)  Indices=1  OutputSizes=1
  Constant : Constant  Value=FLT_ERRBIT_51
  Data Store Read : DataStoreRead  DataStoreName=Flt_ErrCode  IndexOptions=Index vector (dialog)  Indices=1  OutputSizes=1
  Data Store Write : DataStoreWrite  DataStoreName=Flt_ErrCode  IndexOptions=Index vector (dialog)  Indices=1  OutputSizes=1
  wires:
  Data Store Read/1 -> Assignment/1
  Assignment/1 -> Data Store Write/1
  ErrCod/1 -> Assignment/2
  Constant/1 -> Assignment/3

== system FaultCheck/FaultDiag_HighTask_100us/FltDetn/OverCurrDetn/Flt_IvOverCurrDetn/ErrDetn1/If Action Subsystem ==
  Action Port : ActionPort
  Constant : Constant  Value=FLT_NOERR
  DetnFlg : Outport
  wires:
  Constant/1 -> DetnFlg/1

== system FaultCheck/FaultDiag_HighTask_100us/FltDetn/OverCurrDetn/Flt_IvOverCurrDetn/ErrDetn1/If Action Subsystem1 ==
  InputVal : Inport
  ErrDeb : Inport  Port=2
  UpLimPositv : Inport  Port=3
  UpLimNegatv : Inport  Port=4
  Action Port : ActionPort
  Constant3 : Constant  Value=FLT_ERR
  Debounce1 : Subsystem
  Delay1 : Delay  DelayLength=1
  OR : Logic  Operator=OR  AllPortsSameDT=off  OutDataTypeStr=boolean
  Relational Operator : RelationalOperator  Operator=<=  OutDataTypeStr=boolean  RndMeth=Simplest  InputSameDT=off
  Relational Operator1 : RelationalOperator  OutDataTypeStr=boolean  RndMeth=Simplest  InputSameDT=off
  Switch2 : Switch  Criteria=u2 > Threshold  SaturateOnIntegerOverflow=off  InputSameDT=off
  DetnFlg : Outport  PortDimensions=1
  wires:
  InputVal/1 -> Relational Operator1/1, Relational Operator/1
  Relational Operator/1 -> OR/2
  Relational Operator1/1 -> OR/1
  UpLimPositv/1 -> Relational Operator1/2
  OR/1 -> Debounce1/1(ErrInput)  "vvvv_c"
  UpLimNegatv/1 -> Relational Operator/2
  Delay1/1 -> Switch2/3
  Constant3/1 -> Switch2/1
  Switch2/1 -> Delay1/1, DetnFlg/1
  Debounce1/1(ErrFlg) -> Switch2/2
  ErrDeb/1 -> Debounce1/2(ErrDeb)

== system FaultCheck/FaultDiag_HighTask_100us/FltDetn/OverCurrDetn/Flt_IvOverCurrDetn/FltLvl/If Action Subsystem ==
  Action Port : ActionPort
  Constant : Constant  Value=FLTLVL_ZERO
  ValOut : Outport
  wires:
  Constant/1 -> ValOut/1

== system FaultCheck/FaultDiag_HighTask_100us/FltDetn/OverCurrDetn/Flt_IvOverCurrDetn/FltLvl/If Action Subsystem1 ==
  In : Inport
  Action Port : ActionPort
  ValOut : Outport
  wires:
  In/1 -> ValOut/1

== system FaultCheck/FaultDiag_HighTask_100us/FltDetn/OverCurrDetn/Flt_IvOverCurrDetn/Power Reduction Coefficient/If Action Subsystem ==
  Action Port : ActionPort
  Constant1 : Constant  Value=FLT_COEF_ONE
  PowRecCoefOut : Outport
  wires:
  Constant1/1 -> PowRecCoefOut/1

== system FaultCheck/FaultDiag_HighTask_100us/FltDetn/OverCurrDetn/Flt_IvOverCurrDetn/Power Reduction Coefficient/If Action Subsystem1 ==
  PowRecCoef : Inport
  Action Port : ActionPort
  PowRecCoefOut : Outport
  wires:
  PowRecCoef/1 -> PowRecCoefOut/1

== system FaultCheck/FaultDiag_HighTask_100us/FltDetn/OverCurrDetn/Flt_IvOverCurrDetn/Power Reduction Coefficient/If Action Subsystem2 ==
  Action Port : ActionPort
  Constant1 : Constant  Value=FLT_COEF_ZERO
  PowRecCoefOut : Outport
  wires:
  Constant1/1 -> PowRecCoefOut/1

== system FaultCheck/FaultDiag_HighTask_100us/FltDetn/OverCurrDetn/Flt_IwOverCurrDetn1/ErrCode1/If Action Subsystem ==
  Action Port : ActionPort
  Assignment : Assignment  IndexMode=Zero-based  DiagnosticForDimensions=Warning  IndexOptions=Index vector (port)  Indices=1  OutputSizes=1
  Constant : Constant  Value=FLT_ERRCODE_0
  Constant1 : Constant  Value=FLT_ERRBIT_51
  Data Store Read : DataStoreRead  DataStoreName=Flt_ErrCode  IndexOptions=Index vector (dialog)  Indices=1  OutputSizes=1
  Data Store Write : DataStoreWrite  DataStoreName=Flt_ErrCode  IndexOptions=Index vector (dialog)  Indices=1  OutputSizes=1
  wires:
  Constant1/1 -> Assignment/3
  Data Store Read/1 -> Assignment/1
  Constant/1 -> Assignment/2
  Assignment/1 -> Data Store Write/1

== system FaultCheck/FaultDiag_HighTask_100us/FltDetn/OverCurrDetn/Flt_IwOverCurrDetn1/ErrCode1/If Action Subsystem1 ==
  ErrCod : Inport
  Action Port : ActionPort
  Assignment : Assignment  IndexMode=Zero-based  DiagnosticForDimensions=Warning  IndexOptions=Index vector (port)  Indices=1  OutputSizes=1
  Constant : Constant  Value=FLT_ERRBIT_51
  Data Store Read : DataStoreRead  DataStoreName=Flt_ErrCode  IndexOptions=Index vector (dialog)  Indices=1  OutputSizes=1
  Data Store Write : DataStoreWrite  DataStoreName=Flt_ErrCode  IndexOptions=Index vector (dialog)  Indices=1  OutputSizes=1
  wires:
  Data Store Read/1 -> Assignment/1
  Assignment/1 -> Data Store Write/1
  ErrCod/1 -> Assignment/2
  Constant/1 -> Assignment/3

== system FaultCheck/FaultDiag_HighTask_100us/FltDetn/OverCurrDetn/Flt_IwOverCurrDetn1/ErrDetn1/If Action Subsystem ==
  Action Port : ActionPort
  Constant : Constant  Value=FLT_NOERR
  DetnFlg : Outport
  wires:
  Constant/1 -> DetnFlg/1

== system FaultCheck/FaultDiag_HighTask_100us/FltDetn/OverCurrDetn/Flt_IwOverCurrDetn1/ErrDetn1/If Action Subsystem1 ==
  InputVal : Inport
  ErrDeb : Inport  Port=2
  UpLimPositv : Inport  Port=3
  UpLimNegatv : Inport  Port=4
  Action Port : ActionPort
  Constant3 : Constant  Value=FLT_ERR
  Debounce1 : Subsystem
  Delay1 : Delay  DelayLength=1
  OR : Logic  Operator=OR  AllPortsSameDT=off  OutDataTypeStr=boolean
  Relational Operator : RelationalOperator  Operator=<=  OutDataTypeStr=boolean  RndMeth=Simplest  InputSameDT=off
  Relational Operator1 : RelationalOperator  OutDataTypeStr=boolean  RndMeth=Simplest  InputSameDT=off
  Switch2 : Switch  Criteria=u2 > Threshold  SaturateOnIntegerOverflow=off  InputSameDT=off
  DetnFlg : Outport  PortDimensions=1
  wires:
  InputVal/1 -> Relational Operator1/1, Relational Operator/1
  Relational Operator/1 -> OR/2  "w2_C"
  Relational Operator1/1 -> OR/1  "w1_C"
  UpLimPositv/1 -> Relational Operator1/2
  OR/1 -> Debounce1/1(ErrInput)  "wwww_C"
  UpLimNegatv/1 -> Relational Operator/2
  Delay1/1 -> Switch2/3
  Constant3/1 -> Switch2/1
  Switch2/1 -> Delay1/1, DetnFlg/1
  Debounce1/1(ErrFlg) -> Switch2/2
  ErrDeb/1 -> Debounce1/2(ErrDeb)

== system FaultCheck/FaultDiag_HighTask_100us/FltDetn/OverCurrDetn/Flt_IwOverCurrDetn1/FltLvl/If Action Subsystem ==
  Action Port : ActionPort
  Constant : Constant  Value=FLTLVL_ZERO
  ValOut : Outport
  wires:
  Constant/1 -> ValOut/1

== system FaultCheck/FaultDiag_HighTask_100us/FltDetn/OverCurrDetn/Flt_IwOverCurrDetn1/FltLvl/If Action Subsystem1 ==
  In : Inport
  Action Port : ActionPort
  ValOut : Outport
  wires:
  In/1 -> ValOut/1

== system FaultCheck/FaultDiag_HighTask_100us/FltDetn/OverCurrDetn/Flt_IwOverCurrDetn1/Power Reduction Coefficient/If Action Subsystem ==
  Action Port : ActionPort
  Constant1 : Constant  Value=FLT_COEF_ONE
  PowRecCoefOut : Outport
  wires:
  Constant1/1 -> PowRecCoefOut/1

== system FaultCheck/FaultDiag_HighTask_100us/FltDetn/OverCurrDetn/Flt_IwOverCurrDetn1/Power Reduction Coefficient/If Action Subsystem1 ==
  PowRecCoef : Inport
  Action Port : ActionPort
  PowRecCoefOut : Outport
  wires:
  PowRecCoef/1 -> PowRecCoefOut/1

== system FaultCheck/FaultDiag_HighTask_100us/FltDetn/OverCurrDetn/Flt_IwOverCurrDetn1/Power Reduction Coefficient/If Action Subsystem2 ==
  Action Port : ActionPort
  Constant1 : Constant  Value=FLT_COEF_ZERO
  PowRecCoefOut : Outport
  wires:
  Constant1/1 -> PowRecCoefOut/1

== system FaultCheck/FaultDiag_HighTask_100us/FltDetn/RecUDetn/RecUDetn/ErrCode1/If Action Subsystem ==
  Action Port : ActionPort
  Assignment : Assignment  IndexMode=Zero-based  DiagnosticForDimensions=Warning  IndexOptions=Index vector (port)  Indices=1  OutputSizes=1
  Constant : Constant  Value=FLT_ERRCODE_0  OutDataTypeStr=fixdt('uint16', 'DataTypeOverride', 'Off')
  Constant1 : Constant  Value=FLT_ERRBIT_75
  Data Store Read : DataStoreRead  DataStoreName=Flt_ErrCode  IndexOptions=Index vector (dialog)  Indices=1  OutputSizes=1
  Data Store Write : DataStoreWrite  DataStoreName=Flt_ErrCode  IndexOptions=Index vector (dialog)  Indices=1  OutputSizes=1
  wires:
  Assignment/1 -> Data Store Write/1
  Constant/1 -> Assignment/2
  Data Store Read/1 -> Assignment/1
  Constant1/1 -> Assignment/3

== system FaultCheck/FaultDiag_HighTask_100us/FltDetn/RecUDetn/RecUDetn/ErrCode1/If Action Subsystem1 ==
  ErrCod : Inport
  Action Port : ActionPort
  Assignment : Assignment  IndexMode=Zero-based  DiagnosticForDimensions=Warning  IndexOptions=Index vector (port)  Indices=1  OutputSizes=1
  Constant : Constant  Value=FLT_ERRBIT_75
  Data Store Read : DataStoreRead  DataStoreName=Flt_ErrCode  IndexOptions=Index vector (dialog)  Indices=1  OutputSizes=1
  Data Store Write : DataStoreWrite  DataStoreName=Flt_ErrCode  IndexOptions=Index vector (dialog)  Indices=1  OutputSizes=1
  wires:
  Constant/1 -> Assignment/3
  ErrCod/1 -> Assignment/2
  Assignment/1 -> Data Store Write/1
  Data Store Read/1 -> Assignment/1

== system FaultCheck/FaultDiag_HighTask_100us/FltDetn/RecUDetn/RecUDetn/ErrDetn/If Action Subsystem ==
  Action Port : ActionPort
  Constant : Constant  Value=FLT_NOERR
  Out1 : Outport
  wires:
  Constant/1 -> Out1/1

== system FaultCheck/FaultDiag_HighTask_100us/FltDetn/RecUDetn/RecUDetn/ErrDetn/If Action Subsystem1 ==
  InputVal : Inport
  ErrDeb : Inport  Port=2
  Action Port : ActionPort
  Constant3 : Constant  Value=FLT_ERR
  Debounce : Subsystem
  Delay1 : Delay  DelayLength=1
  Signal Conversion : SignalConversion  OverrideOpt=off
  Switch2 : Switch  Criteria=u2 > Threshold  SaturateOnIntegerOverflow=off  InputSameDT=off
  Out1 : Outport
  wires:
  Signal Conversion/1 -> Out1/1
  ErrDeb/1 -> Debounce/2(ErrDeb)
  InputVal/1 -> Debounce/1(ErrInput)
  Debounce/1(ErrFlg) -> Switch2/2
  Switch2/1 -> Delay1/1, Signal Conversion/1
  Constant3/1 -> Switch2/1
  Delay1/1 -> Switch2/3

== system FaultCheck/FaultDiag_HighTask_100us/FltDetn/RecUDetn/RecUDetn/FltLvl/If Action Subsystem ==
  Action Port : ActionPort
  Constant : Constant  Value=FLTLVL_ZERO
  ValOut : Outport
  wires:
  Constant/1 -> ValOut/1

== system FaultCheck/FaultDiag_HighTask_100us/FltDetn/RecUDetn/RecUDetn/FltLvl/If Action Subsystem1 ==
  In : Inport
  Action Port : ActionPort
  ValOut : Outport
  wires:
  In/1 -> ValOut/1

== system FaultCheck/FaultDiag_HighTask_100us/FltDetn/RecUDetn/RecUDetn/Power Reduction Coefficient/If Action Subsystem ==
  Action Port : ActionPort
  Constant1 : Constant  Value=FLT_COEF_ONE
  PowRecCoefOut : Outport
  wires:
  Constant1/1 -> PowRecCoefOut/1

== system FaultCheck/FaultDiag_HighTask_100us/FltDetn/RecUDetn/RecUDetn/Power Reduction Coefficient/If Action Subsystem1 ==
  PowRecCoef : Inport
  Action Port : ActionPort
  PowRecCoefOut : Outport
  wires:
  PowRecCoef/1 -> PowRecCoefOut/1

== system FaultCheck/FaultDiag_HighTask_100us/FltDetn/RecUDetn/RecUDetn/Power Reduction Coefficient/If Action Subsystem2 ==
  Action Port : ActionPort
  Constant1 : Constant  Value=FLT_COEF_ZERO
  PowRecCoefOut : Outport
  wires:
  Constant1/1 -> PowRecCoefOut/1

== system FaultCheck/FaultDiag_HighTask_100us/FltDetn/ResErrFlgDetn/ResErrDetn/ErrCode/If Action Subsystem ==
  Action Port : ActionPort
  Assignment : Assignment  IndexMode=Zero-based  DiagnosticForDimensions=Warning  IndexOptions=Index vector (port)  Indices=1  OutputSizes=1
  Constant : Constant  Value=FLT_ERRCODE_0
  Constant1 : Constant  Value=FLT_ERRBIT_70
  Data Store Read : DataStoreRead  DataStoreName=Flt_ErrCode  IndexOptions=Index vector (dialog)  Indices=1  OutputSizes=1
  Data Store Write : DataStoreWrite  DataStoreName=Flt_ErrCode  IndexOptions=Index vector (dialog)  Indices=1  OutputSizes=1
  wires:
  Constant1/1 -> Assignment/3
  Data Store Read/1 -> Assignment/1
  Constant/1 -> Assignment/2
  Assignment/1 -> Data Store Write/1

== system FaultCheck/FaultDiag_HighTask_100us/FltDetn/ResErrFlgDetn/ResErrDetn/ErrCode/If Action Subsystem1 ==
  ErrCod : Inport
  Action Port : ActionPort
  Assignment : Assignment  IndexMode=Zero-based  DiagnosticForDimensions=Warning  IndexOptions=Index vector (port)  Indices=1  OutputSizes=1
  Constant : Constant  Value=FLT_ERRBIT_70
  Data Store Read : DataStoreRead  DataStoreName=Flt_ErrCode  IndexOptions=Index vector (dialog)  Indices=1  OutputSizes=1
  Data Store Write : DataStoreWrite  DataStoreName=Flt_ErrCode  IndexOptions=Index vector (dialog)  Indices=1  OutputSizes=1
  wires:
  Data Store Read/1 -> Assignment/1
  Assignment/1 -> Data Store Write/1
  ErrCod/1 -> Assignment/2
  Constant/1 -> Assignment/3

== system FaultCheck/FaultDiag_HighTask_100us/FltDetn/ResErrFlgDetn/ResErrDetn/ErrDetn/If Action Subsystem ==
  Action Port : ActionPort
  Constant : Constant  Value=FLT_NOERR
  Out1 : Outport
  wires:
  Constant/1 -> Out1/1

== system FaultCheck/FaultDiag_HighTask_100us/FltDetn/ResErrFlgDetn/ResErrDetn/ErrDetn/If Action Subsystem1 ==
  InputVal : Inport
  Action Port : ActionPort
  Constant3 : Constant  Value=FLT_ERR
  Delay1 : Delay  DelayLength=1
  Switch2 : Switch  Criteria=u2 > Threshold  SaturateOnIntegerOverflow=off  InputSameDT=off
  Out1 : Outport
  wires:
  InputVal/1 -> Switch2/2
  Switch2/1 -> Delay1/1, Out1/1
  Constant3/1 -> Switch2/1
  Delay1/1 -> Switch2/3

== system FaultCheck/FaultDiag_HighTask_100us/FltDetn/ResErrFlgDetn/ResErrDetn/FltLvl/If Action Subsystem ==
  Action Port : ActionPort
  Constant : Constant  Value=FLTLVL_ZERO
  ValOut : Outport
  wires:
  Constant/1 -> ValOut/1

== system FaultCheck/FaultDiag_HighTask_100us/FltDetn/ResErrFlgDetn/ResErrDetn/FltLvl/If Action Subsystem1 ==
  In : Inport
  Action Port : ActionPort
  ValOut : Outport
  wires:
  In/1 -> ValOut/1

== system FaultCheck/FaultDiag_HighTask_100us/FltDetn/ResErrFlgDetn/ResErrDetn/Power Reduction Coefficient/If Action Subsystem ==
  Action Port : ActionPort
  Constant1 : Constant  Value=FLT_COEF_ONE
  PowRecCoefOut : Outport
  wires:
  Constant1/1 -> PowRecCoefOut/1

== system FaultCheck/FaultDiag_HighTask_100us/FltDetn/ResErrFlgDetn/ResErrDetn/Power Reduction Coefficient/If Action Subsystem1 ==
  PowRecCoef : Inport
  Action Port : ActionPort
  PowRecCoefOut : Outport
  wires:
  PowRecCoef/1 -> PowRecCoefOut/1

== system FaultCheck/FaultDiag_HighTask_100us/FltDetn/ResErrFlgDetn/ResErrDetn/Power Reduction Coefficient/If Action Subsystem2 ==
  Action Port : ActionPort
  Constant1 : Constant  Value=FLT_COEF_ZERO
  PowRecCoefOut : Outport
  wires:
  Constant1/1 -> PowRecCoefOut/1

== system FaultCheck/FaultDiag_HighTask_100us/FltDetn/ResolveSensorDetn/Flt_ResolveSensorDetn/ErrCode/If Action Subsystem ==
  Action Port : ActionPort
  Assignment : Assignment  IndexMode=Zero-based  DiagnosticForDimensions=Warning  IndexOptions=Index vector (port)  Indices=1  OutputSizes=1
  Constant : Constant  Value=FLT_ERRCODE_0  OutDataTypeStr=fixdt('uint16', 'DataTypeOverride', 'Off')
  Constant1 : Constant  Value=FLT_ERRBIT_53
  Data Store Read : DataStoreRead  DataStoreName=Flt_ErrCode  IndexOptions=Index vector (dialog)  Indices=1  OutputSizes=1
  Data Store Write : DataStoreWrite  DataStoreName=Flt_ErrCode  IndexOptions=Index vector (dialog)  Indices=1  OutputSizes=1
  wires:
  Assignment/1 -> Data Store Write/1
  Constant/1 -> Assignment/2
  Data Store Read/1 -> Assignment/1
  Constant1/1 -> Assignment/3

== system FaultCheck/FaultDiag_HighTask_100us/FltDetn/ResolveSensorDetn/Flt_ResolveSensorDetn/ErrCode/If Action Subsystem1 ==
  ErrCod : Inport
  Action Port : ActionPort
  Assignment : Assignment  IndexMode=Zero-based  DiagnosticForDimensions=Warning  IndexOptions=Index vector (port)  Indices=1  OutputSizes=1
  Constant : Constant  Value=FLT_ERRBIT_53
  Data Store Read : DataStoreRead  DataStoreName=Flt_ErrCode  IndexOptions=Index vector (dialog)  Indices=1  OutputSizes=1
  Data Store Write : DataStoreWrite  DataStoreName=Flt_ErrCode  IndexOptions=Index vector (dialog)  Indices=1  OutputSizes=1
  wires:
  Constant/1 -> Assignment/3
  ErrCod/1 -> Assignment/2
  Assignment/1 -> Data Store Write/1
  Data Store Read/1 -> Assignment/1

== system FaultCheck/FaultDiag_HighTask_100us/FltDetn/ResolveSensorDetn/Flt_ResolveSensorDetn/ErrDetn/If Action Subsystem ==
  Action Port : ActionPort
  Constant : Constant  Value=FLT_NOERR
  Out1 : Outport
  wires:
  Constant/1 -> Out1/1

== system FaultCheck/FaultDiag_HighTask_100us/FltDetn/ResolveSensorDetn/Flt_ResolveSensorDetn/ErrDetn/If Action Subsystem1 ==
  InputVal : Inport
  ErrDeb : Inport  Port=2
  Action Port : ActionPort
  Constant3 : Constant  Value=FLT_ERR
  Debounce1 : Subsystem
  Delay1 : Delay  DelayLength=1
  Signal Conversion : SignalConversion  OverrideOpt=off
  Switch2 : Switch  Criteria=u2 > Threshold  SaturateOnIntegerOverflow=off  InputSameDT=off
  Out1 : Outport
  wires:
  Signal Conversion/1 -> Out1/1
  Delay1/1 -> Switch2/3
  Constant3/1 -> Switch2/1
  Switch2/1 -> Signal Conversion/1, Delay1/1
  Debounce1/1(ErrFlg) -> Switch2/2
  InputVal/1 -> Debounce1/1(ErrInput)
  ErrDeb/1 -> Debounce1/2(ErrDeb)

== system FaultCheck/FaultDiag_HighTask_100us/FltDetn/ResolveSensorDetn/Flt_ResolveSensorDetn/FltLvl/If Action Subsystem ==
  Action Port : ActionPort
  Constant : Constant  Value=FLTLVL_ZERO
  ValOut : Outport
  wires:
  Constant/1 -> ValOut/1

== system FaultCheck/FaultDiag_HighTask_100us/FltDetn/ResolveSensorDetn/Flt_ResolveSensorDetn/FltLvl/If Action Subsystem1 ==
  In : Inport
  Action Port : ActionPort
  ValOut : Outport
  wires:
  In/1 -> ValOut/1

== system FaultCheck/FaultDiag_HighTask_100us/FltDetn/ResolveSensorDetn/Flt_ResolveSensorDetn/Power Reduction Coefficient/If Action Subsystem ==
  Action Port : ActionPort
  Constant1 : Constant  Value=FLT_COEF_ONE
  PowRecCoefOut : Outport
  wires:
  Constant1/1 -> PowRecCoefOut/1
